simulink model "Ident_friccion_step1_GB2"  (Simulink 6.6)
settings: Solver=ode4  StartTime=0.0  StopTime=20  RelTol=1e-3
PreLoadFcn:
  | inicializacion_step1
StopFcn:
  | saveDATA_Ident_friccion_STEP1_GB
values from neighbouring files (symbols this model uses):
  K1 = 1.1    [inicializacion_step1.m]
  K2 = 1.1    [inicializacion_step1.m]
  precision = precisiones(7)    [inicializacion_step1.m]
  tau = 0.001    [inicializacion_step1.m]    (also in preparacion_datos_step1.m)
  tau1 = 0.1    [inicializacion_step1.m]
  tau2 = 0.05    [inicializacion_step1.m]
  w1 = 4    [inicializacion_step1.m]
  w2 = 4    [inicializacion_step1.m]
  zero_c = 1500    [inicializacion_step1.m]
  zero_h = 200    [inicializacion_step1.m]
libraries: simulink x7, xpcnilib x4, xpclib x4
settings Model: Creator=BEJARANO_ROBOT2GDL  LastModifiedBy=BEJARANO_ROBOT2GDL  SimulationMode=external  ExtModeArmWhenConnect=off  BufferReuse=off
settings OptimizationCC: BlockReduction=off  OptimizeBlockIOStorage=off  BufferReuse=off  ExpressionFolding=off  FoldNonRolledExpr=off  LocalBlockOutputs=off
settings DebuggingCC: SignalResolutionControl=TryResolveAllWithWarning  MultiTaskDSMMsg=warning  MultiTaskCondExecSysMsg=none  StrictBusMsg=None
settings RTWCC: SystemTargetFile=xpctarget.tlc  TemplateMakefile=xpc_default_tmf  Description=xPC Target  ProcessScript=xpctarget_make_rtw_hook  IncludeERTFirstTime=on
settings xpcTargetCC: TargetFcnLib=ansi_tfl_tmw.mat  GenFloatMathFcnCalls=ANSI_C  PortableWordSizes=off  RL32LogBufSizeModifier=10000000

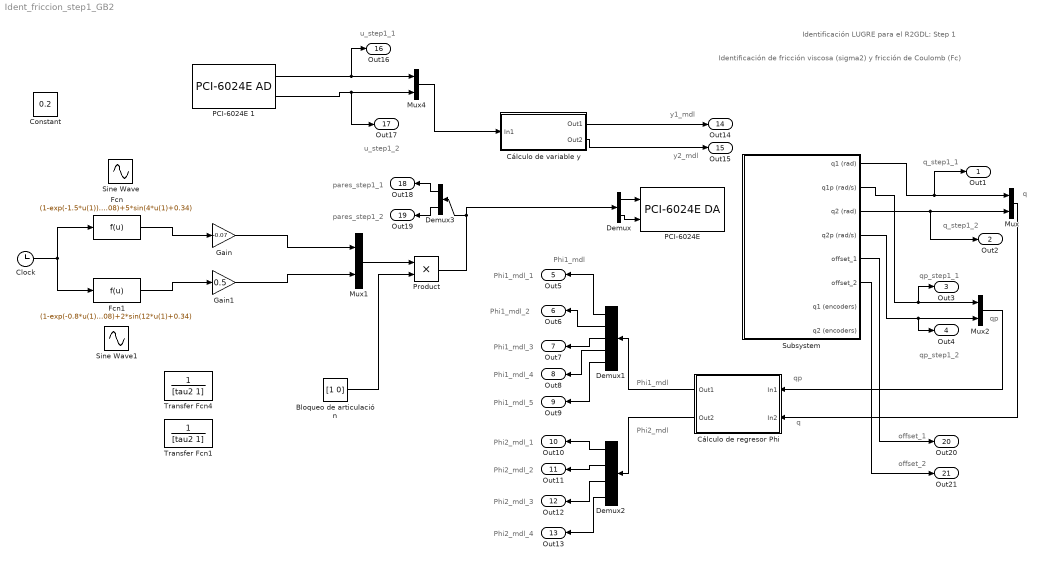
== system Ident_friccion_step1_GB2 ==
  note: q
  note: qp
  note: qp
  note: q
  note: qp_step1_1
  note: Phi1_mdl
  note: Phi2_mdl
  note: y1_mdl
  note: y2_mdl
  note: Identificación LUGRE para el R2GDL: Step 1
  note: Identificación de fricción viscosa (sigma2) y fricción de Coulomb (Fc)
  note: u_step1_1
  note: q_step1_1
  note: q_step1_2
  note: qp_step1_2
  note: Phi1_mdl
  note: Phi1_mdl_2
  note: Phi1_mdl_1
  note: Phi1_mdl_3
  note: Phi1_mdl_4
  note: Phi1_mdl_5
  note: Phi2_mdl_1
  note: Phi2_mdl_2
  note: Phi2_mdl_3
  note: Phi2_mdl_4
  note: u_step1_2
  note: pares_step1_1
  note: pares_step1_2
  note: offset_1
  note: offset_2
  Bloqueo de articulación : Constant  Value=[1 0]
  Clock : Clock
      settings: Decimation=10
  Cálculo de regresor Phi : Subsystem  Orientation=left
  Cálculo de variable y : Subsystem
  Demux : Demux  Outputs=2
  Demux1 : Demux  Orientation=left  Outputs=5
  Demux2 : Demux  Orientation=left
  Demux3 : Demux  Orientation=left  Outputs=2
  Fcn : Fcn  Expr=(1-exp(-1.5*u(1)))*5+8*sin(8*u(1)+0.08)+5*sin(4*u(1)+0.34)
  Fcn1 : Fcn  Expr=(1-exp(-0.8*u(1)))*1.2+8*sin(26*u(1)+0.08)+2*sin(12*u(1)+0.34)
  Gain : Gain  Gain=-0.07
  Gain1 : Gain  Gain=0.5
  Mux{,1..2,4} (4 alike) : Mux  Inputs=2
  "PCI-6024E " : xpcnilib/D//A/PCI-6024E DA  channel=[1,2]  reset=[1]  initValue=[0]  sampletime=0.001  slot=-1
  PCI-6024E 1 : xpcnilib/A//D/PCI-6024E AD  channel=[3,4]  range=[-10,-10]  coupling=[0,0]  sampletime=0.001  slot=-1
  Product : Product  RndMeth=Zero
  Sine Wave : Sin  Amplitude=K1  Frequency=w1  SampleTime=0
  Sine Wave1 : Sin  Amplitude=K2  Frequency=w2  SampleTime=0
  Subsystem : Subsystem
  Transfer Fcn1 : TransferFcn  Denominator=[tau2 1]
  Transfer Fcn4 : TransferFcn  Denominator=[tau2 1]
  Out1 : Outport
  Out2 : Outport  Port=2
  Out3 : Outport  Port=3
  Out4 : Outport  Port=4
  Out5 : Outport  Orientation=left  Port=5
  Out6 : Outport  Orientation=left  Port=6
  Out7 : Outport  Orientation=left  Port=7
  Out8 : Outport  Orientation=left  Port=8
  Out9 : Outport  Orientation=left  Port=9
  Out10 : Outport  Orientation=left  Port=10
  Out11 : Outport  Orientation=left  Port=11
  Out12 : Outport  Orientation=left  Port=12
  Out13 : Outport  Orientation=left  Port=13
  Out14 : Outport  Port=14
  Out15 : Outport  Port=15
  Out16 : Outport  Port=16
  Out17 : Outport  Port=17
  Out18 : Outport  Orientation=left  Port=18
  Out19 : Outport  Orientation=left  Port=19
  Out20 : Outport  Port=20
  Out21 : Outport  Port=21
  Constant : Constant  IOType=siggen  Value=0.2
  wires:
  Bloqueo de articulación/1 -> Product/2
  Mux1/1 -> Product/1
  Product/1 -> Demux/1, Demux3/1
  Mux/1 -> Cálculo de regresor Phi/2(In2)
  Subsystem/2(q1p (rad/s)) -> Mux2/1, Out3/1
  Subsystem/4(q2p (rad/s)) -> Mux2/2, Out4/1
  Mux2/1 -> Cálculo de regresor Phi/1(In1)
  Demux/1 -> "PCI-6024E "/1
  Demux/2 -> "PCI-6024E "/2
  Cálculo de regresor Phi/1(Out1) -> Demux1/1
  Cálculo de regresor Phi/2(Out2) -> Demux2/1
  Cálculo de variable y/1(Out1) -> Out14/1
  Cálculo de variable y/2(Out2) -> Out15/1
  Mux4/1 -> Cálculo de variable y/1(In1)
  PCI-6024E 1/1 -> Mux4/1, Out16/1
  PCI-6024E 1/2 -> Mux4/2, Out17/1
  Subsystem/3(q2 (rad)) -> Mux/2, Out2/1
  Demux1/1 -> Out5/1
  Demux1/2 -> Out6/1
  Demux1/3 -> Out7/1
  Demux1/4 -> Out8/1
  Demux1/5 -> Out9/1
  Demux2/1 -> Out10/1
  Demux2/2 -> Out11/1
  Demux2/3 -> Out12/1
  Demux2/4 -> Out13/1
  Demux3/1 -> Out18/1
  Demux3/2 -> Out19/1
  Subsystem/1(q1 (rad)) -> Out1/1, Mux/1
  Subsystem/5(offset_1) -> Out20/1
  Subsystem/6(offset_2) -> Out21/1
  Clock/1 -> Fcn/1, Fcn1/1
  Fcn1/1 -> Gain1/1
  Fcn/1 -> Gain/1
  Gain/1 -> Mux1/1
  Gain1/1 -> Mux1/2

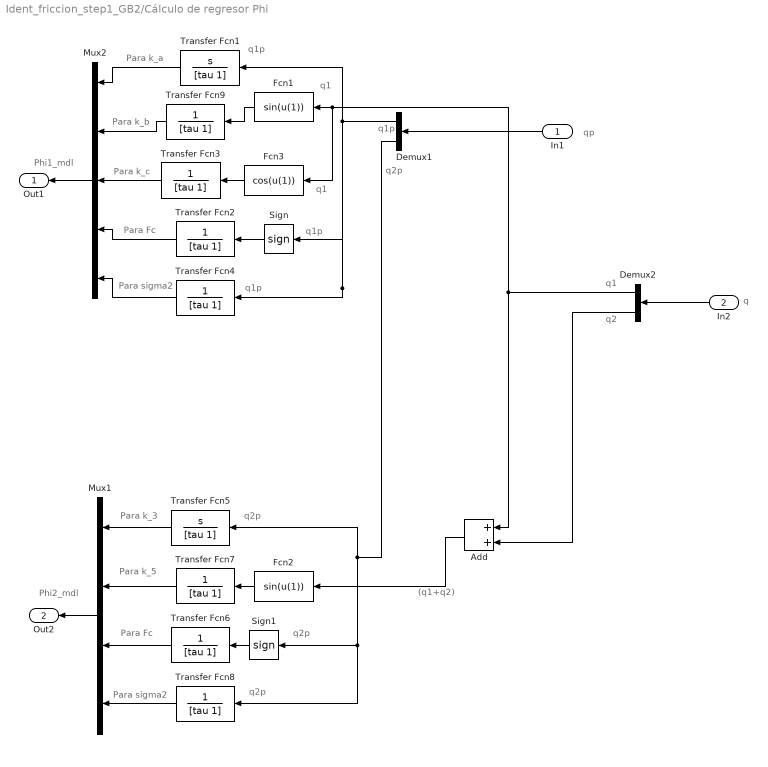
== system Ident_friccion_step1_GB2/Cálculo de regresor Phi ==
  note: q1
  note: q1p
  note: q1p
  note: q1p
  note: q1
  note: q1p
  note: q2p
  note: q2p
  note: q2p
  note: q2p
  note: q1
  note: q2
  note: (q1+q2)
  note: qp
  note: q
  note: Para k_a
  note: Para k_b
  note: Para k_c
  note: Para Fc
  note: Para sigma2
  note: Para k_3
  note: Para k_5
  note: Para Fc
  note: Para sigma2
  note: Phi1_mdl
  note: Phi2_mdl
  In1 : Inport  Orientation=left
  In2 : Inport  Orientation=left  Port=2
  Add : Sum  Orientation=left  OutScaling=2^-10
  Demux1 : Demux  Orientation=left  Outputs=2
  Demux2 : Demux  Orientation=left  Outputs=2
  Fcn1 : Fcn  Orientation=left  Expr=sin(u(1))
  Fcn2 : Fcn  Orientation=left  Expr=sin(u(1))
  Fcn3 : Fcn  Orientation=left  Expr=cos(u(1))
  Mux1 : Mux  Orientation=left
  Mux2 : Mux  Orientation=left  Inputs=5
  Sign : Signum  Orientation=left
  Sign1 : Signum  Orientation=left
  Transfer Fcn1 : TransferFcn  Orientation=left  Numerator=[1 0]  Denominator=[tau 1]
  Transfer Fcn{2..4,6..9} (7 alike) : TransferFcn  Orientation=left  Denominator=[tau 1]
  Transfer Fcn5 : TransferFcn  Orientation=left  Numerator=[1 0]  Denominator=[tau 1]
  Out1 : Outport  Orientation=left
  Out2 : Outport  Orientation=left  Port=2
  wires:
  Transfer Fcn1/1 -> Mux2/1
  Sign/1 -> Transfer Fcn2/1
  Demux1/1 -> Transfer Fcn1/1, Transfer Fcn4/1, Sign/1
  Mux2/1 -> Out1/1
  In1/1 -> Demux1/1
  Demux1/2 -> Transfer Fcn5/1, Transfer Fcn8/1, Sign1/1
  Transfer Fcn5/1 -> Mux1/1
  Transfer Fcn7/1 -> Mux1/2
  Fcn2/1 -> Transfer Fcn7/1
  Sign1/1 -> Transfer Fcn6/1
  Transfer Fcn6/1 -> Mux1/3
  Transfer Fcn8/1 -> Mux1/4
  Mux1/1 -> Out2/1
  In2/1 -> Demux2/1
  Demux2/1 -> Add/1, Fcn1/1, Fcn3/1
  Demux2/2 -> Add/2
  Add/1 -> Fcn2/1
  Transfer Fcn4/1 -> Mux2/5
  Transfer Fcn2/1 -> Mux2/4
  Fcn3/1 -> Transfer Fcn3/1
  Transfer Fcn3/1 -> Mux2/3
  Fcn1/1 -> Transfer Fcn9/1
  Transfer Fcn9/1 -> Mux2/2

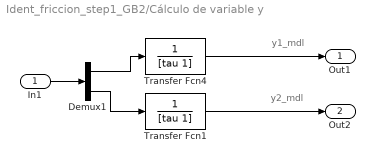
== system Ident_friccion_step1_GB2/Cálculo de variable y ==
  note: y1_mdl
  note: y2_mdl
  In1 : Inport
  Demux1 : Demux  Outputs=2
  Transfer Fcn1 : TransferFcn  Denominator=[tau 1]
  Transfer Fcn4 : TransferFcn  Denominator=[tau 1]
  Out1 : Outport
  Out2 : Outport  Port=2
  wires:
  Demux1/1 -> Transfer Fcn4/1
  Demux1/2 -> Transfer Fcn1/1
  Transfer Fcn1/1 -> Out2/1
  In1/1 -> Demux1/1
  Transfer Fcn4/1 -> Out1/1

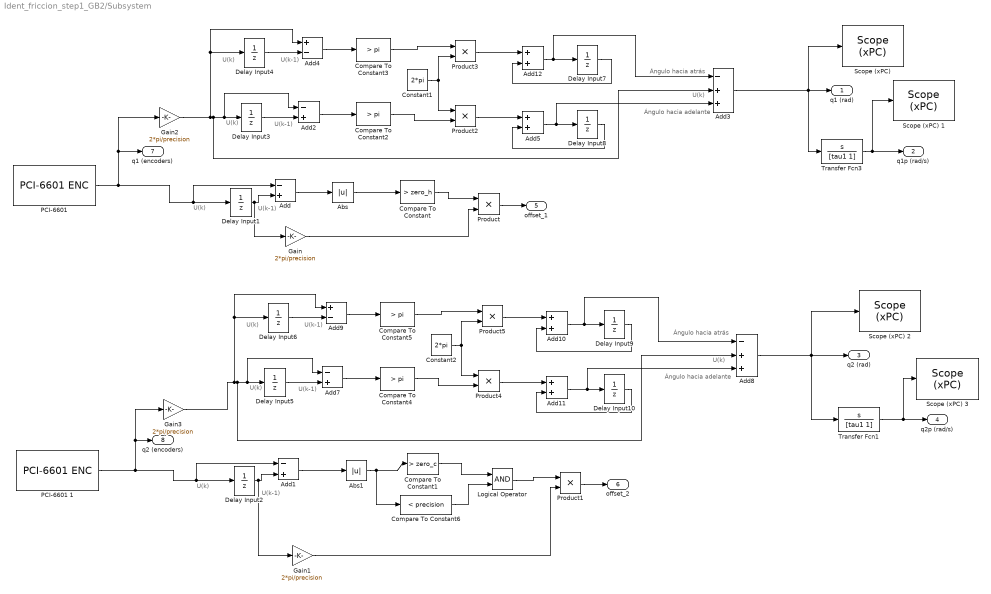
== system Ident_friccion_step1_GB2/Subsystem ==
  note: U(k)
  note: U(k)
  note: U(k-1)
  note: U(k-1)
  note: U(k)
  note: U(k-1)
  note: U(k-1)
  note: U(k)
  note: U(k)
  note: Ángulo hacia atrás
  note: Ángulo hacia adelante
  note: U(k)
  note: U(k-1)
  note: U(k-1)
  note: U(k)
  note: U(k)
  note: Ángulo hacia atrás
  note: Ángulo hacia adelante
  Abs : Abs
  Abs1 : Abs
  Add{,1..2,7} (4 alike) : Sum  Inputs=-+  OutScaling=2^-10
  Add{5,10..12} (4 alike) : Sum  OutScaling=2^-10
  Add3 : Sum  Inputs=-++  OutScaling=2^-10
  Add4 : Sum  Inputs=+-  OutScaling=2^-10
  Add8 : Sum  Inputs=-++  OutScaling=2^-10
  Add9 : Sum  Inputs=+-  OutScaling=2^-10
  Compare To Constant : simulink/Logic and Bit Operations/Compare To Constant  SystemSampleTime=-1  relop=>  const=zero_h  LogicOutDataTypeMode=uint8  ZeroCross=off
  Compare To Constant1 : simulink/Logic and Bit Operations/Compare To Constant  SystemSampleTime=-1  relop=>  const=zero_c  LogicOutDataTypeMode=uint8  ZeroCross=off
  Compare To Constant{2..5} (4 alike) : simulink/Logic and Bit Operations/Compare To Constant  SystemSampleTime=-1  relop=>  const=pi  LogicOutDataTypeMode=uint8  ZeroCross=off
  Compare To Constant6 : simulink/Logic and Bit Operations/Compare To Constant  SystemSampleTime=-1  relop=<  const=precision  LogicOutDataTypeMode=uint8  ZeroCross=off
  Constant1 : Constant  Value=2*pi
  Constant2 : Constant  Value=2*pi
  Delay Input{1..10} (10 alike) : UnitDelay  Description=Store in Global RAM  SampleTime=-1
  Gain{,1..3} (4 alike) : Gain  Gain=2*pi/precision
  Logical Operator : Logic  AllPortsSameDT=off  OutDataTypeMode=Specify via dialog
  "PCI-6601 " : xpcnilib/Incremental Encoder/PCI-6601 ENC  channel=1  countMode=Quadrature Mode X1  initCount=0  reload=on  indexPhase=A high B high  filter=None  sampleTime=0.001  slot=-1
  PCI-6601 1 : xpcnilib/Incremental Encoder/PCI-6601 ENC  channel=2  countMode=Quadrature Mode X1  initCount=0  reload=on  indexPhase=A high B high  filter=None  sampleTime=0.001  slot=-1
  Product{,1..5} (6 alike) : Product  RndMeth=Zero
  "Scope (xPC) " : xpclib/Misc./Scope (xPC)   SystemSampleTime=-1  scopeno=1  scopetype=Target  autostart=on  viewmode=Graphical redraw  formatstr='%15.6f'  grid=on  ylimits=[0,0]  nosamples=250  noprepostsamples=0  interleave=1  triggermode=FreeRun  triggersignal=1  triggerlevel=0.0  triggerslope=Either  triggerscope=1  triggersample=0  filename=data.dat  mode=Lazy  writesize=512  autorestart=off
  Scope (xPC) 1 : xpclib/Misc./Scope (xPC)   SystemSampleTime=-1  scopeno=2  scopetype=Target  autostart=on  viewmode=Graphical redraw  formatstr='%15.6f'  grid=on  ylimits=[0,0]  nosamples=250  noprepostsamples=0  interleave=1  triggermode=FreeRun  triggersignal=1  triggerlevel=0.0  triggerslope=Either  triggerscope=1  triggersample=0  filename=data.dat  mode=Lazy  writesize=512  autorestart=off
  Scope (xPC) 2 : xpclib/Misc./Scope (xPC)   SystemSampleTime=-1  scopeno=3  scopetype=Target  autostart=on  viewmode=Graphical redraw  formatstr='%15.6f'  grid=on  ylimits=[0,0]  nosamples=250  noprepostsamples=0  interleave=1  triggermode=FreeRun  triggersignal=1  triggerlevel=0.0  triggerslope=Either  triggerscope=1  triggersample=0  filename=data.dat  mode=Lazy  writesize=512  autorestart=off
  Scope (xPC) 3 : xpclib/Misc./Scope (xPC)   SystemSampleTime=-1  scopeno=4  scopetype=Target  autostart=on  viewmode=Graphical redraw  formatstr='%15.6f'  grid=on  ylimits=[0,0]  nosamples=250  noprepostsamples=0  interleave=1  triggermode=FreeRun  triggersignal=1  triggerlevel=0.0  triggerslope=Either  triggerscope=1  triggersample=0  filename=data.dat  mode=Lazy  writesize=512  autorestart=off
  Transfer Fcn1 : TransferFcn  Numerator=[1 0]  Denominator=[tau1 1]
  Transfer Fcn3 : TransferFcn  Numerator=[1 0]  Denominator=[tau1 1]
  q1 (rad) : Outport
  q1p (rad/s) : Outport  Port=2
  q2 (rad) : Outport  Port=3
  q2p (rad/s) : Outport  Port=4
  offset_1 : Outport  Port=5
  offset_2 : Outport  Port=6
  q1 (encoders) : Outport  Port=7
  q2 (encoders) : Outport  Port=8
  wires:
  "PCI-6601 "/1 -> Gain2/1, q1 (encoders)/1, Delay Input1/1, Add/1
  Delay Input1/1 -> Add/2, Gain/1
  Compare To Constant/1 -> Product/1
  Gain/1 -> Product/2
  Delay Input2/1 -> Add1/2, Gain1/1
  Gain1/1 -> Product1/2
  PCI-6601 1/1 -> Add1/1, Delay Input2/1, Gain3/1, q2 (encoders)/1
  Product/1 -> offset_1/1
  Product1/1 -> offset_2/1
  Add/1 -> Abs/1
  Abs/1 -> Compare To Constant/1
  Add1/1 -> Abs1/1
  Abs1/1 -> Compare To Constant1/1, Compare To Constant6/1
  Delay Input3/1 -> Add2/2
  Gain2/1 -> Delay Input4/1, Add4/1, Add2/1, Delay Input3/1, Add3/2
  Add2/1 -> Compare To Constant2/1
  Compare To Constant2/1 -> Product2/2
  Transfer Fcn3/1 -> q1p (rad/s)/1, Scope (xPC) 1/1
  Delay Input4/1 -> Add4/2
  Add4/1 -> Compare To Constant3/1
  Compare To Constant3/1 -> Product3/1
  Constant1/1 -> Product3/2, Product2/1
  Add3/1 -> q1 (rad)/1, "Scope (xPC) "/1, Transfer Fcn3/1
  Delay Input5/1 -> Add7/2
  Gain3/1 -> Delay Input6/1, Add9/1, Add7/1, Delay Input5/1, Add8/2
  Add7/1 -> Compare To Constant4/1
  Compare To Constant4/1 -> Product4/2
  Delay Input6/1 -> Add9/2
  Add9/1 -> Compare To Constant5/1
  Compare To Constant5/1 -> Product5/1
  Product5/1 -> Add10/1
  Product4/1 -> Add11/1
  Transfer Fcn1/1 -> q2p (rad/s)/1, Scope (xPC) 3/1
  Add8/1 -> q2 (rad)/1, Scope (xPC) 2/1, Transfer Fcn1/1
  Delay Input7/1 -> Add12/2
  Add12/1 -> Delay Input7/1, Add3/1
  Product3/1 -> Add12/1
  Product2/1 -> Add5/1
  Add5/1 -> Delay Input8/1, Add3/3
  Delay Input8/1 -> Add5/2
  Add10/1 -> Delay Input9/1, Add8/1
  Add11/1 -> Delay Input10/1, Add8/3
  Delay Input10/1 -> Add11/2
  Delay Input9/1 -> Add10/2
  Compare To Constant1/1 -> Logical Operator/1
  Compare To Constant6/1 -> Logical Operator/2
  Logical Operator/1 -> Product1/1
  Constant2/1 -> Product5/2, Product4/1
